simulink model "ssc_pneumatic_actuator"  (R2021b)
settings: Solver=VariableStepAuto  StartTime=0.0  StopTime=10.0  RelTol=1e-3  AbsTol=1e-3
PreLoadFcn:
  | delta_p = 0.6; % MPa
  | p_init = 0.101325; % MPa
  | T_init = 293.15; % K
  | T_atm = 293.15; % K
  | 
  | A_valve_max = 4e-6; % m^2
  | A_valve_min = 1e-10; % m^2
  | 
  | A_pipe = 5e-6; % m^2
  | L_pipe = 1; % m
  | 
  | A_piston = 0.002; % m^2
  | L_piston = 0.2; % m
undefined symbols (not defined in the file): sigbuilder_block
libraries: fl_lib x49, nesl_utility x3
(part 2 of 2)

== system ssc_pneumatic_actuator/Atm ==
  Temperature Source : fl_lib/Thermal/Thermal Sources/Temperature Source  temperature=T_atm K
  T : PMIOPort  Side=Right
  connections:
  Temperature Source/LConn1 -- T/RConn1

== system ssc_pneumatic_actuator/Atm1 ==
  Temperature Source : fl_lib/Thermal/Thermal Sources/Temperature Source  temperature=T_atm K
  T : PMIOPort  Side=Right
  connections:
  Temperature Source/LConn1 -- T/RConn1

== system ssc_pneumatic_actuator/Atm2 ==
  Temperature Source : fl_lib/Thermal/Thermal Sources/Temperature Source  temperature=T_atm K
  T : PMIOPort  Side=Right
  connections:
  Temperature Source/LConn1 -- T/RConn1

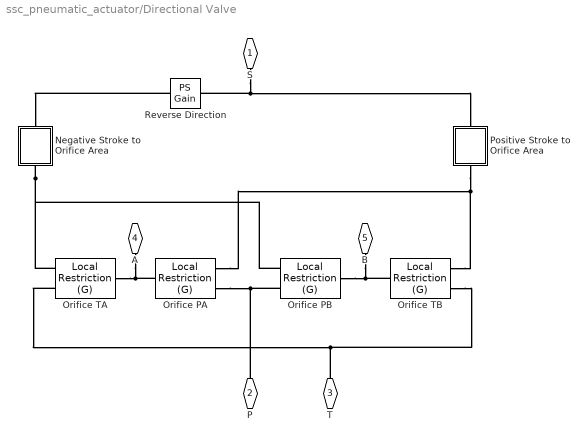
== system ssc_pneumatic_actuator/Directional Valve ==
  Negative Stroke to Orifice Area : Subsystem
  Orifice PA : fl_lib/Gas/Elements/Local Restriction (G)  restriction_type=foundation.enum.restriction_type.variable  restriction_area=1e-3 m^2  min_area=A_leakage m^2  max_area=A_max m^2  area=A_port m^2  Cd=Cd  B_lam=0.999
      settings: SourceProductBaseCode=SS  InternalSimscapePortConfiguration="{\"Bottom\":[],\"Left\":[{\"id\":\"A\",\"label\":\"A\",\"type\":\"foundation.gas.gas\"},{\"id\":\"area_in\",\"label\":\"AR\",\"type\":\"input\"}],\"Right\":[{\"id\":\"B\",\"label\":\"B\",\"type\":\"foundation.gas.gas\"}],\"Top\":[]}"
  Orifice PB : fl_lib/Gas/Elements/Local Restriction (G)  restriction_type=foundation.enum.restriction_type.variable  restriction_area=1e-3 m^2  min_area=A_leakage m^2  max_area=A_max m^2  area=A_port m^2  Cd=Cd  B_lam=0.999
      settings: SourceProductBaseCode=SS  InternalSimscapePortConfiguration="{\"Bottom\":[],\"Left\":[{\"id\":\"A\",\"label\":\"A\",\"type\":\"foundation.gas.gas\"},{\"id\":\"area_in\",\"label\":\"AR\",\"type\":\"input\"}],\"Right\":[{\"id\":\"B\",\"label\":\"B\",\"type\":\"foundation.gas.gas\"}],\"Top\":[]}"
  Orifice TA : fl_lib/Gas/Elements/Local Restriction (G)  restriction_type=foundation.enum.restriction_type.variable  restriction_area=1e-3 m^2  min_area=A_leakage m^2  max_area=A_max m^2  area=A_port m^2  Cd=Cd  B_lam=0.999
      settings: SourceProductBaseCode=SS  InternalSimscapePortConfiguration="{\"Bottom\":[],\"Left\":[{\"id\":\"A\",\"label\":\"A\",\"type\":\"foundation.gas.gas\"},{\"id\":\"area_in\",\"label\":\"AR\",\"type\":\"input\"}],\"Right\":[{\"id\":\"B\",\"label\":\"B\",\"type\":\"foundation.gas.gas\"}],\"Top\":[]}"
  Orifice TB : fl_lib/Gas/Elements/Local Restriction (G)  restriction_type=foundation.enum.restriction_type.variable  restriction_area=1e-3 m^2  min_area=A_leakage m^2  max_area=A_max m^2  area=A_port m^2  Cd=Cd  B_lam=0.999
      settings: SourceProductBaseCode=SS  InternalSimscapePortConfiguration="{\"Bottom\":[],\"Left\":[{\"id\":\"A\",\"label\":\"A\",\"type\":\"foundation.gas.gas\"},{\"id\":\"area_in\",\"label\":\"AR\",\"type\":\"input\"}],\"Right\":[{\"id\":\"B\",\"label\":\"B\",\"type\":\"foundation.gas.gas\"}],\"Top\":[]}"
  Positive Stroke to Orifice Area : Subsystem
  Reverse Direction : fl_lib/Physical Signals/Functions/PS Gain  gain=-1
  S : PMIOPort  Side=Left
  P : PMIOPort  Port=2  Side=Left
  T : PMIOPort  Port=3  Side=Left
  A : PMIOPort  Port=4  Side=Right
  B : PMIOPort  Port=5  Side=Right
  connections:
  B/RConn1 -- Orifice TB/RConn1 -- Orifice PB/RConn1
  A/RConn1 -- Orifice PA/RConn1 -- Orifice TA/RConn1
  T/RConn1 -- Orifice TB/LConn1 -- Orifice TA/LConn1
  P/RConn1 -- Orifice PB/LConn1 -- Orifice PA/LConn1
  S/RConn1 -- Positive Stroke to Orifice Area/LConn1 -- Reverse Direction/LConn1
  Positive Stroke to Orifice Area/RConn1 -- Orifice TB/LConn2 -- Orifice PA/LConn2
  Negative Stroke to Orifice Area/RConn1 -- Orifice PB/LConn2 -- Orifice TA/LConn2
  Reverse Direction/RConn1 -- Negative Stroke to Orifice Area/LConn1

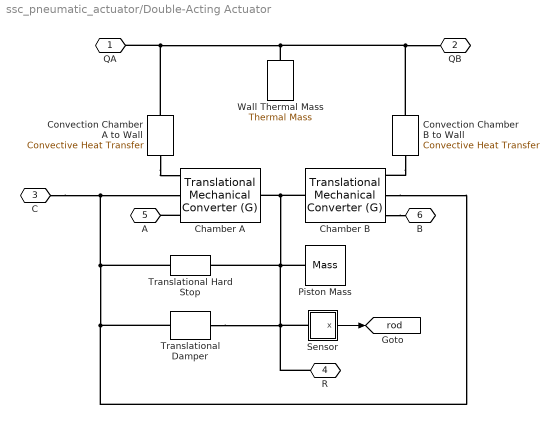
== system ssc_pneumatic_actuator/Double-Acting Actuator ==
  Chamber A : fl_lib/Gas/Elements/Translational Mechanical Converter (G)  mech_orientation=simscape.enum.posneg.positive  displacement_spec=foundation.enum.DisplacementSpec.Calculate  length_init=x_init m  interface_area=A_piston m^2  dead_volume=0.1 * A_piston * x_max m^3  area_A=A_port m^2  environment_spec=foundation.enum.pressure_spec.atmospheric  environment_pressure=0.101325 MPa  p_I_specify=on  p_I_priority=High  p_I=p_init MPa  p_I_nominal_specify=off  p_I_nominal_unit=MPa  p_I_nominal_value=1  T_I_specify=on  T_I_priority=High  T_I=T_init K  T_I_nominal_specify=off  T_I_nominal_unit=K  T_I_nominal_value=1  rho_converter_specify=off  rho_converter_priority=None  rho_converter=1.2 kg/m^3  rho_converter_nominal_specify=off  rho_converter_nominal_unit=kg/m^3  rho_converter_nominal_value=1
      settings: SourceProductBaseCode=SS  InternalSimscapePortConfiguration="{\"Bottom\":[],\"Left\":[{\"id\":\"A\",\"label\":\"A\",\"type\":\"foundation.gas.gas\"},{\"id\":\"C\",\"label\":\"C\",\"type\":\"foundation.mechanical.translational.translational\"},{\"id\":\"H\",\"label\":\"H\",\"type\":\"foundation.thermal.thermal\"}],\"Right\":[{\"id\":\"R\",\"label\":\"R\",\"type\":\"foundation.mechanical.translational.translational\"}],\"Top\":[]}"
  Chamber B : fl_lib/Gas/Elements/Translational Mechanical Converter (G)  mech_orientation=simscape.enum.posneg.negative  displacement_spec=foundation.enum.DisplacementSpec.Calculate  length_init=- x_max + x_init m  interface_area=A_piston m^2  dead_volume=0.1 * A_piston * x_max m^3  area_A=A_port m^2  environment_spec=foundation.enum.pressure_spec.atmospheric  environment_pressure=0.101325 MPa  p_I_specify=on  p_I_priority=High  p_I=p_init MPa  p_I_nominal_specify=off  p_I_nominal_unit=MPa  p_I_nominal_value=1  T_I_specify=on  T_I_priority=High  T_I=T_init K  T_I_nominal_specify=off  T_I_nominal_unit=K  T_I_nominal_value=1  rho_converter_specify=off  rho_converter_priority=None  rho_converter=1.2 kg/m^3  rho_converter_nominal_specify=off  rho_converter_nominal_unit=kg/m^3  rho_converter_nominal_value=1
      settings: SourceProductBaseCode=SS  InternalSimscapePortConfiguration="{\"Bottom\":[],\"Left\":[{\"id\":\"A\",\"label\":\"A\",\"type\":\"foundation.gas.gas\"},{\"id\":\"C\",\"label\":\"C\",\"type\":\"foundation.mechanical.translational.translational\"},{\"id\":\"H\",\"label\":\"H\",\"type\":\"foundation.thermal.thermal\"}],\"Right\":[{\"id\":\"R\",\"label\":\"R\",\"type\":\"foundation.mechanical.translational.translational\"}],\"Top\":[]}"
  Convection Chamber A to Wall : fl_lib/Thermal/Thermal Elements/Convective Heat Transfer  area=2*A_piston + sqrt(pi*A_piston)*x_max m^2  heat_tr_coeff=heat_coeff W/(m^2 * K)  T_specify=off  T_priority=None  T=0 K  T_nominal_specify=off  T_nominal_unit=K  T_nominal_value=1  Q_specify=off  Q_priority=None  Q=0 W  Q_nominal_specify=off  Q_nominal_unit=W  Q_nominal_value=1
  Convection Chamber B to Wall : fl_lib/Thermal/Thermal Elements/Convective Heat Transfer  area=2*A_piston + sqrt(pi*A_piston)*x_max m^2  heat_tr_coeff=heat_coeff W/(m^2 * K)  T_specify=off  T_priority=None  T=0 K  T_nominal_specify=off  T_nominal_unit=K  T_nominal_value=1  Q_specify=off  Q_priority=None  Q=0 W  Q_nominal_specify=off  Q_nominal_unit=W  Q_nominal_value=1
  Piston Mass : fl_lib/Mechanical/Translational Elements/Mass  mass=M_piston kg  num_ports=foundation.enum.numPorts2.one  v_specify=off  v_priority=High  v=0 m/s  v_nominal_specify=off  v_nominal_unit=m/s  v_nominal_value=1  f_specify=off  f_priority=None  f=0 N  f_nominal_specify=off  f_nominal_unit=N  f_nominal_value=1
  Sensor : Subsystem
      mask Display: disp('S')
  Translational Damper : fl_lib/Mechanical/Translational Elements/Translational Damper  D=damp_mech N/(m/s)  v_specify=off  v_priority=None  v=0 m/s  v_nominal_specify=off  v_nominal_unit=m/s  v_nominal_value=1  f_specify=off  f_priority=None  f=0 N  f_nominal_specify=off  f_nominal_unit=N  f_nominal_value=1
  Translational Hard Stop : fl_lib/Mechanical/Translational Elements/Translational Hard Stop  upper_bnd=x_max m  lower_bnd=0 m  stiff_up=stiff_hard_stop N/m  stiff_low=stiff_hard_stop N/m  D_up=damp_hard_stop N/(m/s)  D_low=damp_hard_stop N/(m/s)  model=3  transition=0.1 mm  v_specify=off  v_priority=None  v=0 m/s  v_nominal_specify=off  v_nominal_unit=m/s  v_nominal_value=1  f_specify=off  f_priority=None  f=0 N  f_nominal_specify=off  f_nominal_unit=N  f_nominal_value=1  x_specify=on  x_priority=High  x=x_init m  x_nominal_specify=off  x_nominal_unit=m  x_nominal_value=1
  Wall Thermal Mass : fl_lib/Thermal/Thermal Elements/Thermal Mass  mass=M_actuator kg  sp_heat=cp J/kg/K  T_specify=on  T_priority=High  T=T_init K  T_nominal_specify=off  T_nominal_unit=K  T_nominal_value=1  Q_specify=off  Q_priority=None  Q=0 W  Q_nominal_specify=off  Q_nominal_unit=W  Q_nominal_value=1
  QA : PMIOPort  Side=Left
  QB : PMIOPort  Port=2  Side=Right
  C : PMIOPort  Port=3  Side=Left
  R : PMIOPort  Port=4  Side=Right
  A : PMIOPort  Port=5  Side=Left
  B : PMIOPort  Port=6  Side=Right
  tag scope: rod=global
  wires:
  Sensor/1(x) -> [rod]
  connections:
  Chamber B/RConn1 -- R/RConn1 -- Sensor/LConn1 -- Translational Damper/LConn1 -- Piston Mass/LConn1 -- Translational Hard Stop/LConn1 -- Chamber A/RConn1
  Convection Chamber A to Wall/RConn1 -- QA/RConn1 -- Wall Thermal Mass/LConn1 -- Convection Chamber B to Wall/RConn1 -- QB/RConn1
  Translational Hard Stop/RConn1 -- Chamber B/LConn2 -- Translational Damper/RConn1 -- C/RConn1 -- Chamber A/LConn2
  Chamber A/LConn1 -- A/RConn1
  Chamber B/LConn1 -- B/RConn1
  Convection Chamber A to Wall/LConn1 -- Chamber A/LConn3
  Convection Chamber B to Wall/LConn1 -- Chamber B/LConn3

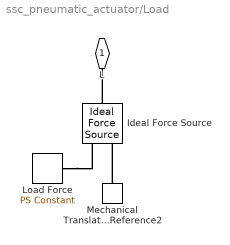
== system ssc_pneumatic_actuator/Load ==
  Ideal Force Source : fl_lib/Mechanical/Mechanical Sources/Ideal Force Source
  Load Force : fl_lib/Physical Signals/Sources/PS Constant  constant=-500 N
  Mechanical Translational Reference2 : fl_lib/Mechanical/Translational Elements/Mechanical Translational Reference
  L : PMIOPort  Side=Right
  connections:
  Load Force/RConn1 -- Ideal Force Source/RConn1
  Mechanical Translational Reference2/LConn1 -- Ideal Force Source/RConn2
  Ideal Force Source/LConn1 -- L/RConn1

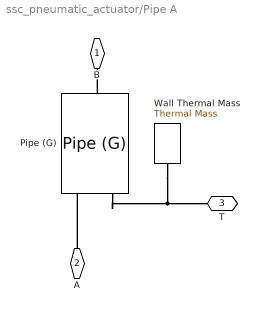
== system ssc_pneumatic_actuator/Pipe A ==
  Pipe (G) : fl_lib/Gas/Elements/Pipe (G)  length=L_pipe m  area=A_pipe m^2  Dh=2*sqrt(A_pipe/pi) m  length_add=0.1 * L_pipe m  roughness=15e-6 m  Re_lam=2000  Re_tur=4000  shape_factor=64  Nu_lam=3.66  p_I_specify=on  p_I_priority=High  p_I=p_init MPa  p_I_nominal_specify=off  p_I_nominal_unit=MPa  p_I_nominal_value=1  T_I_specify=on  T_I_priority=High  T_I=T_init K  T_I_nominal_specify=off  T_I_nominal_unit=K  T_I_nominal_value=1  rho_pipe_specify=off  rho_pipe_priority=None  rho_pipe=1.2 kg/m^3  rho_pipe_nominal_specify=off  rho_pipe_nominal_unit=kg/m^3  rho_pipe_nominal_value=1
      settings: SourceProductBaseCode=SS
  Wall Thermal Mass : fl_lib/Thermal/Thermal Elements/Thermal Mass  mass=rho_wall * A_pipe * L_pipe kg  sp_heat=cp_wall J/kg/K  T_specify=on  T_priority=High  T=T_init K  T_nominal_specify=off  T_nominal_unit=K  T_nominal_value=1  Q_specify=off  Q_priority=None  Q=0 W  Q_nominal_specify=off  Q_nominal_unit=W  Q_nominal_value=1
  B : PMIOPort  Side=Right
  A : PMIOPort  Port=2  Side=Left
  T : PMIOPort  Port=3  Side=Left
  connections:
  Pipe (G)/RConn1 -- B/RConn1
  A/RConn1 -- Pipe (G)/LConn1
  Pipe (G)/LConn2 -- Wall Thermal Mass/LConn1 -- T/RConn1

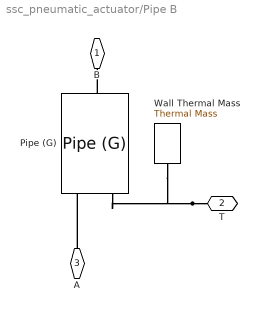
== system ssc_pneumatic_actuator/Pipe B ==
  Pipe (G) : fl_lib/Gas/Elements/Pipe (G)  length=L_pipe m  area=A_pipe m^2  Dh=2*sqrt(A_pipe/pi) m  length_add=0.1 * L_pipe m  roughness=15e-6 m  Re_lam=2000  Re_tur=4000  shape_factor=64  Nu_lam=3.66  p_I_specify=on  p_I_priority=High  p_I=p_init MPa  p_I_nominal_specify=off  p_I_nominal_unit=MPa  p_I_nominal_value=1  T_I_specify=on  T_I_priority=High  T_I=T_init K  T_I_nominal_specify=off  T_I_nominal_unit=K  T_I_nominal_value=1  rho_pipe_specify=off  rho_pipe_priority=None  rho_pipe=1.2 kg/m^3  rho_pipe_nominal_specify=off  rho_pipe_nominal_unit=kg/m^3  rho_pipe_nominal_value=1
      settings: SourceProductBaseCode=SS
  Wall Thermal Mass : fl_lib/Thermal/Thermal Elements/Thermal Mass  mass=rho_wall * A_pipe * L_pipe kg  sp_heat=cp_wall J/kg/K  T_specify=on  T_priority=High  T=T_init K  T_nominal_specify=off  T_nominal_unit=K  T_nominal_value=1  Q_specify=off  Q_priority=None  Q=0 W  Q_nominal_specify=off  Q_nominal_unit=W  Q_nominal_value=1
  B : PMIOPort  Side=Right
  T : PMIOPort  Port=2  Side=Left
  A : PMIOPort  Port=3  Side=Left
  connections:
  T/RConn1 -- Wall Thermal Mass/LConn1 -- Pipe (G)/LConn2
  A/RConn1 -- Pipe (G)/LConn1
  Pipe (G)/RConn1 -- B/RConn1

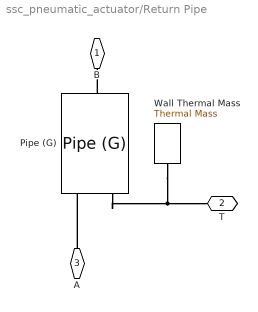
== system ssc_pneumatic_actuator/Return Pipe ==
  Pipe (G) : fl_lib/Gas/Elements/Pipe (G)  length=L_pipe m  area=A_pipe m^2  Dh=2*sqrt(A_pipe/pi) m  length_add=0.1 * L_pipe m  roughness=15e-6 m  Re_lam=2000  Re_tur=4000  shape_factor=64  Nu_lam=3.66  p_I_specify=on  p_I_priority=High  p_I=p_init MPa  p_I_nominal_specify=off  p_I_nominal_unit=MPa  p_I_nominal_value=1  T_I_specify=on  T_I_priority=High  T_I=T_init K  T_I_nominal_specify=off  T_I_nominal_unit=K  T_I_nominal_value=1  rho_pipe_specify=off  rho_pipe_priority=None  rho_pipe=1.2 kg/m^3  rho_pipe_nominal_specify=off  rho_pipe_nominal_unit=kg/m^3  rho_pipe_nominal_value=1
      settings: SourceProductBaseCode=SS
  Wall Thermal Mass : fl_lib/Thermal/Thermal Elements/Thermal Mass  mass=rho_wall * A_pipe * L_pipe kg  sp_heat=cp_wall J/kg/K  T_specify=on  T_priority=High  T=T_init K  T_nominal_specify=off  T_nominal_unit=K  T_nominal_value=1  Q_specify=off  Q_priority=None  Q=0 W  Q_nominal_specify=off  Q_nominal_unit=W  Q_nominal_value=1
  B : PMIOPort  Side=Right
  T : PMIOPort  Port=2  Side=Left
  A : PMIOPort  Port=3  Side=Left
  connections:
  Pipe (G)/RConn1 -- B/RConn1
  A/RConn1 -- Pipe (G)/LConn1
  Pipe (G)/LConn2 -- Wall Thermal Mass/LConn1 -- T/RConn1

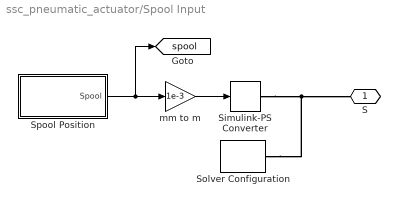
== system ssc_pneumatic_actuator/Spool Input ==
  Simulink-PS Converter : nesl_utility/Simulink-PS Converter  PhysicalDomain=network_engine_domain  SubClassName=ps_input  LeftPortType=input  RightPortType=output  PseudoPeriodic=off  Frequencies=[]  NoiseDistribution=none  NoiseParameters=[]  Unit=m  AffineConversion=off  FilteringAndDerivatives=zero  SimscapeFilterOrder=1  InputFilterTimeConstant=0.001  UdotUserProvided=1
      settings: SourceProductBaseCode=PW,SS
  Solver Configuration : nesl_utility/Solver Configuration  PhysicalDomain=network_engine_domain  SubClassName=solver  LeftPortType=input  RightPortType=generic  Tones=[]  Harmonics=[]  SimulateNoise=off  Profile=off  UseLocalSampling=off  EnableSwitchedLinearOptims=on  FrequencyDomain=off  UseCCode=off  RelTol=0.001  AbsTol=1e-06  MinStep=1e-09  ToWorkspace=off  RevertToSquareIcSolve=off  NumHomotopyIterations=100  PhasorMode=off  PhasorModeNumHarmonics=1  DoDC=off  ResidualTolerance=1e-9  UseLocalSolver=off  LocalSolverChoice=NE_BACKWARD_EULER_ADVANCER  LocalSolverSampleTime=0.001  DoFixedCost=off  MaxNonlinIter=3  MaxModeIter=2  ComputeImpulses=off  ImpulseIterations=2  LinearAlgebra=auto  EquationFormulation=NE_TIME_EF  DelaysMemoryBudget=1024  AutomaticFiltering=on  FilteringTimeConstant=0.001  PartitionStorageMethod=AS_NEEDED  PartitionMemoryBudget=1024  PartitionMethod=FAST
      settings: SourceProductBaseCode=PW,SS
  Spool Position : Subsystem  Tag=STV Subsys  LoadFcn=sigbuilder_block('load');  StartFcn=sigbuilder_block('start');  StopFcn=sigbuilder_block('stop');  ClipboardFcn=sigbuilder_block('clipboard');  mask(Sigbuilder block){tuvar=[0:10]}
      mask help: Simulink:masks:SigbuilderBlock_MD
      mask init:
      | if ~strcmp(get_param(bdroot(gcbh),'SimulationStatus'),'stopped') tuvar = sigbuilder_block('maskInit'); end
      settings: CopyFcn=sigbuilder_block('copy');  DeleteFcn=sigbuilder_block('delete');  ModelCloseFcn=sigbuilder_block('modelClose');  PreSaveFcn=sigbuilder_block('preSave');  PauseFcn=sigbuilder_block('pause');  ContinueFcn=sigbuilder_block('continue');  NameChangeFcn=sigbuilder_block('namechange');  OpenFcn=sigbuilder_block('open',[405 316.5 550.5 399.75 ]);  CloseFcn=sigbuilder_block('close');
      mask Display: plot(0, 0, 100, 100,[2, 2, 32, 32, 2], [68, 8, 8, 68, 68],[32, 2], [38, 38], [32, 19, 2],[53, 60, 44], [32, 17, 17, 2],[16, 16, 31, 31]);txt = getActiveGroup(gcbh);text(2, 100, txt,'verticalAlignment', 'top');
  mm to m : Gain  Gain=1e-3
  S : PMIOPort  Side=Right
  tag scope: spool=global
  wires:
  Spool Position/1(Spool) -> [spool], mm to m/1
  mm to m/1 -> Simulink-PS Converter/1
  connections:
  Simulink-PS Converter/RConn1 -- S/RConn1 -- Solver Configuration/RConn1

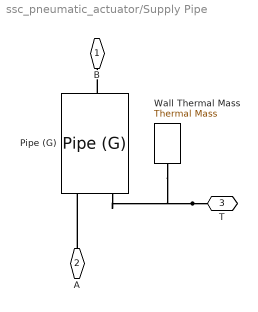
== system ssc_pneumatic_actuator/Supply Pipe ==
  Pipe (G) : fl_lib/Gas/Elements/Pipe (G)  length=L_pipe m  area=A_pipe m^2  Dh=2*sqrt(A_pipe/pi) m  length_add=0.1 * L_pipe m  roughness=15e-6 m  Re_lam=2000  Re_tur=4000  shape_factor=64  Nu_lam=3.66  p_I_specify=on  p_I_priority=High  p_I=p_init MPa  p_I_nominal_specify=off  p_I_nominal_unit=MPa  p_I_nominal_value=1  T_I_specify=on  T_I_priority=High  T_I=T_init K  T_I_nominal_specify=off  T_I_nominal_unit=K  T_I_nominal_value=1  rho_pipe_specify=off  rho_pipe_priority=None  rho_pipe=1.2 kg/m^3  rho_pipe_nominal_specify=off  rho_pipe_nominal_unit=kg/m^3  rho_pipe_nominal_value=1
      settings: SourceProductBaseCode=SS
  Wall Thermal Mass : fl_lib/Thermal/Thermal Elements/Thermal Mass  mass=rho_wall * A_pipe * L_pipe kg  sp_heat=cp_wall J/kg/K  T_specify=on  T_priority=High  T=T_init K  T_nominal_specify=off  T_nominal_unit=K  T_nominal_value=1  Q_specify=off  Q_priority=None  Q=0 W  Q_nominal_specify=off  Q_nominal_unit=W  Q_nominal_value=1
  B : PMIOPort  Side=Right
  A : PMIOPort  Port=2  Side=Left
  T : PMIOPort  Port=3  Side=Left
  connections:
  T/RConn1 -- Wall Thermal Mass/LConn1 -- Pipe (G)/LConn2
  A/RConn1 -- Pipe (G)/LConn1
  Pipe (G)/RConn1 -- B/RConn1

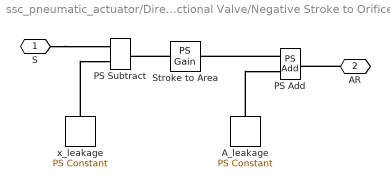
== system ssc_pneumatic_actuator/Directional Valve/Negative Stroke to Orifice Area ==
  A_leakage : fl_lib/Physical Signals/Sources/PS Constant  constant=A_leakage m^2
  PS Add : fl_lib/Physical Signals/Functions/PS Add
  PS Subtract : fl_lib/Physical Signals/Functions/PS Subtract
  Stroke to Area : fl_lib/Physical Signals/Functions/PS Gain  gain=(A_max - A_leakage) / (x_max - x_leakage) m^2/m
  x_leakage : fl_lib/Physical Signals/Sources/PS Constant  constant=x_leakage m
  S : PMIOPort  Side=Left
  AR : PMIOPort  Port=2  Side=Right
  connections:
  S/RConn1 -- PS Subtract/LConn1
  PS Add/LConn1 -- Stroke to Area/RConn1
  Stroke to Area/LConn1 -- PS Subtract/RConn1
  A_leakage/RConn1 -- PS Add/LConn2
  x_leakage/RConn1 -- PS Subtract/LConn2
  AR/RConn1 -- PS Add/RConn1

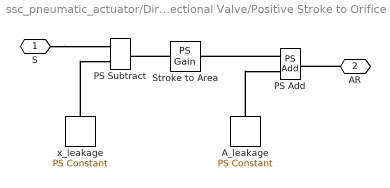
== system ssc_pneumatic_actuator/Directional Valve/Positive Stroke to Orifice Area ==
  A_leakage : fl_lib/Physical Signals/Sources/PS Constant  constant=A_leakage m^2
  PS Add : fl_lib/Physical Signals/Functions/PS Add
  PS Subtract : fl_lib/Physical Signals/Functions/PS Subtract
  Stroke to Area : fl_lib/Physical Signals/Functions/PS Gain  gain=(A_max - A_leakage) / (x_max - x_leakage) m^2/m
  x_leakage : fl_lib/Physical Signals/Sources/PS Constant  constant=x_leakage m
  S : PMIOPort  Side=Left
  AR : PMIOPort  Port=2  Side=Right
  connections:
  AR/RConn1 -- PS Add/RConn1
  x_leakage/RConn1 -- PS Subtract/LConn2
  A_leakage/RConn1 -- PS Add/LConn2
  Stroke to Area/LConn1 -- PS Subtract/RConn1
  PS Add/LConn1 -- Stroke to Area/RConn1
  S/RConn1 -- PS Subtract/LConn1

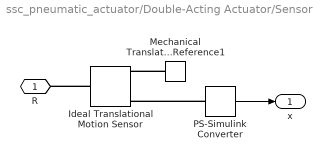
== system ssc_pneumatic_actuator/Double-Acting Actuator/Sensor ==
  Ideal Translational Motion Sensor : fl_lib/Mechanical/Mechanical Sensors/Ideal Translational Motion Sensor  offset=0 m
  Mechanical Translational Reference1 : fl_lib/Mechanical/Translational Elements/Mechanical Translational Reference
  PS-Simulink Converter : nesl_utility/PS-Simulink Converter  PhysicalDomain=network_engine_domain  SubClassName=ps_output  LeftPortType=input  RightPortType=output  PseudoPeriodic=off  Frequencies=[]  Unit=m  AffineConversion=off
      settings: SourceProductBaseCode=PW,SS
  R : PMIOPort  Side=Left
  x : Outport  VectorParamsAs1DForOutWhenUnconnected=off
  wires:
  PS-Simulink Converter/1 -> x/1
  connections:
  Mechanical Translational Reference1/LConn1 -- Ideal Translational Motion Sensor/RConn1
  Ideal Translational Motion Sensor/LConn1 -- R/RConn1
  PS-Simulink Converter/LConn1 -- Ideal Translational Motion Sensor/RConn3

== system ssc_pneumatic_actuator/Spool Input/Spool Position ==
  Demux : Demux  Tag=STV Demux  Outputs=1
      settings: DisplayOption=none
  FromWs : FromWorkspace  Tag=STV FromWs  VariableName=tuvar
      SigBuilderData=|
      | common.afterFinalStr = 'Extrapolate'
      | common.sampleTime = 0
      | dataSet.timeRange = [0 10]
      | dataSet.name = 'Group 1'
      | sbobj.Groups.Name = 'Group 1'
      | sbobj.Groups.Signals.Name = 'Spool'
      | sbobj.Groups.Signals.XData = [0 1 1.2 3.8 4 6 6.2 8.8 9 10]
      | sbobj.Groups.Signals.YData = [0 0 5 5 0 0 -5 -5 0 0]
  Spool : Outport  Tag=STV Outport  VectorParamsAs1DForOutWhenUnconnected=off
  wires:
  Demux/1 -> Spool/1
  FromWs/1 -> Demux/1
